simulink model "ball_bouncing"  (R2017b)
settings: Solver=FixedStepAuto  StartTime=0.0  StopTime=10.0  FixedStep=0.001  RelTol=1e-3
values from neighbouring files (symbols this model uses):
  ba = 25    [ball_bouncing_simulation.m]    (also in init_ball_boucing_simulink.m = 1.8)
  d2xa = diff(dxa)    [impact_equations.m]    (also in init_ball_boucing_simulink.m = 0)
  d2xb = diff(dxb)    [impact_equations.m]    (also in init_ball_boucing_simulink.m = 0)
  dxa = diff(xa)    [impact_equations.m]    (also in init_ball_boucing_simulink.m = 0)
  dxb = diff(xb)    [impact_equations.m]    (also in init_ball_boucing_simulink.m = 0)
  g = 9.81    [ball_bouncing_simulation.m]    (also in init_ball_boucing_simulink.m)
  ka = 500    [ball_bouncing_simulation.m]    (also in init_ball_boucing_simulink.m = 25)
  kb = 15000    [ball_bouncing_simulation.m]    (also in init_ball_boucing_simulink.m = 1500)
  ma = 1    [ball_bouncing_simulation.m]    (also in init_ball_boucing_simulink.m = 0.113)
  mb = 0.058    [ball_bouncing_simulation.m]    (also in init_ball_boucing_simulink.m = 0.025)
  r = 0.05    [ball_bouncing_simulation.m]    (also in init_ball_boucing_simulink.m)
  xa = [xa; y(1:idx_end_impact-1,2)]    [ball_bouncing_simulation.m]    (also in init_ball_boucing_simulink.m = 0)
  xb = [xb; y(1:idx_end_impact-1,1)]    [ball_bouncing_simulation.m]    (also in init_ball_boucing_simulink.m = 0.5)
  xv = 0    [ball_bouncing_simulation.m]    (also in init_ball_boucing_simulink.m)
settings Model: Creator=Vincent  LastModifiedBy=Vincent

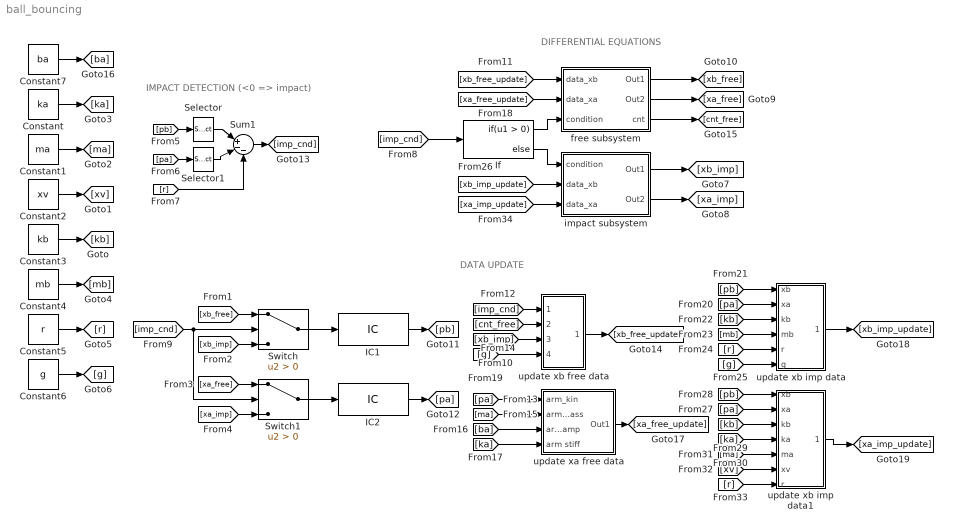
== system ball_bouncing ==
  note: DIFFERENTIAL EQUATIONS
  note: IMPACT DETECTION (<0 => impact)
  note: DATA UPDATE
  Constant : Constant  Value=ka
  Constant1 : Constant  Value=ma
  Constant2 : Constant  Value=xv
  Constant3 : Constant  Value=kb
  Constant4 : Constant  Value=mb
  Constant5 : Constant  Value=r
  Constant6 : Constant  Value=g
  Constant7 : Constant  Value=ba
  IC1 : InitialCondition  Value=[xb;dxb;d2xb]
  IC2 : InitialCondition  Value=[xa;dxa;d2xa]
  If : If
  Selector : Selector  InputPortWidth=3  IndexOptions=Index vector (dialog)  Indices=[1]  OutputSizes=1
  Selector1 : Selector  InputPortWidth=3  IndexOptions=Index vector (dialog)  Indices=[1]  OutputSizes=1
  Sum1 : Sum  Inputs=|+--
  Switch : Switch  Criteria=u2 > Threshold
  Switch1 : Switch  Criteria=u2 > Threshold
  free subsystem : Subsystem
  impact subsystem : Subsystem
  update xa free data : Subsystem
  update xb free data : Subsystem
  update xb imp data : Subsystem
  update xb imp data1 : Subsystem
  wires:
  Constant/1 -> [ka]
  Constant1/1 -> [ma]
  Constant2/1 -> [xv]
  Constant4/1 -> [mb]
  Constant5/1 -> [r]
  Constant6/1 -> [g]
  Constant3/1 -> [kb]
  [imp_cnd] -> If/1
  If/2 -> impact subsystem/1(condition)
  impact subsystem/1(Out1) -> [xb_imp]
  impact subsystem/2(Out2) -> [xa_imp]
  If/1 -> free subsystem/3(condition)
  free subsystem/1(Out1) -> [xb_free]
  free subsystem/2(Out2) -> [xa_free]
  [xb_free] -> Switch/1
  [xb_imp] -> Switch/3
  [xa_free] -> Switch1/1
  [xa_imp] -> Switch1/3
  [pb] -> Selector/1
  Selector/1 -> Sum1/1
  [pa] -> Selector1/1
  Selector1/1 -> Sum1/2
  [r] -> Sum1/3
  Sum1/1 -> [imp_cnd]
  [imp_cnd] -> Switch1/2, Switch/2
  free subsystem/3(cnt) -> [cnt_free]
  [imp_cnd] -> update xb free data/1(In1)
  [cnt_free] -> update xb free data/2(In2)
  [xb_imp] -> update xb free data/3(In3)
  update xb free data/1(Out1) -> [xb_free_update]
  [xb_free_update] -> free subsystem/1(data_xb)
  [pa] -> update xa free data/1(arm_kin)
  [ma] -> update xa free data/2(arm mass)
  [ba] -> update xa free data/3(arm damp)
  [ka] -> update xa free data/4(arm stiff)
  Constant7/1 -> [ba]
  update xa free data/1(Out1) -> [xa_free_update]
  [xa_free_update] -> free subsystem/2(data_xa)
  [g] -> update xb free data/4(In4)
  [pa] -> update xb imp data/2(xa)
  [pb] -> update xb imp data/1(xb)
  [kb] -> update xb imp data/3(kb)
  [mb] -> update xb imp data/4(mb)
  [r] -> update xb imp data/5(r)
  [g] -> update xb imp data/6(g)
  update xb imp data/1(Out1) -> [xb_imp_update]
  [xb_imp_update] -> impact subsystem/2(data_xb)
  update xb imp data1/1(Out1) -> [xa_imp_update]
  [xv] -> update xb imp data1/6(xv)
  [ma] -> update xb imp data1/5(ma)
  [ka] -> update xb imp data1/4(ka)
  [kb] -> update xb imp data1/3(kb)
  [pb] -> update xb imp data1/1(xb)
  [pa] -> update xb imp data1/2(xa)
  [r] -> update xb imp data1/7(r)
  [xa_imp_update] -> impact subsystem/3(data_xa)
  IC2/1 -> [pa]
  Switch/1 -> IC1/1
  IC1/1 -> [pb]
  Switch1/1 -> IC2/1

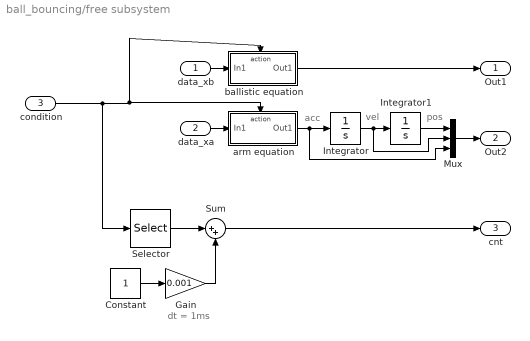
== system ball_bouncing/free subsystem ==
  note: dt = 1ms
  note: acc
  note: pos
  note: vel
  data_xb : Inport
  data_xa : Inport  Port=2
  condition : Inport  Port=3
  Constant : Constant
  Gain : Gain  Gain=0.001
  Integrator : Integrator
  Integrator1 : Integrator
  Mux : Mux  Inputs=3
  Selector : Selector  InputPortWidth=4  IndexOptions=Index vector (dialog)  Indices=[1]  OutputSizes=1
  Sum : Sum  Inputs=|++
  arm equation : Subsystem  TreatAsAtomicUnit=on
  ballistic equation : Subsystem  TreatAsAtomicUnit=on
  Out1 : Outport
  Out2 : Outport  Port=2
  cnt : Outport  Port=3
  wires:
  arm equation/1(Out1) -> Mux/3, Integrator/1
  Integrator/1 -> Mux/2, Integrator1/1
  ballistic equation/1(Out1) -> Out1/1
  condition/1 -> Selector/1, ballistic equation/Action, arm equation/Action
  data_xb/1 -> ballistic equation/1(In1)
  data_xa/1 -> arm equation/1(In1)
  Integrator1/1 -> Mux/1
  Mux/1 -> Out2/1
  Selector/1 -> Sum/1
  Sum/1 -> cnt/1
  Constant/1 -> Gain/1
  Gain/1 -> Sum/2

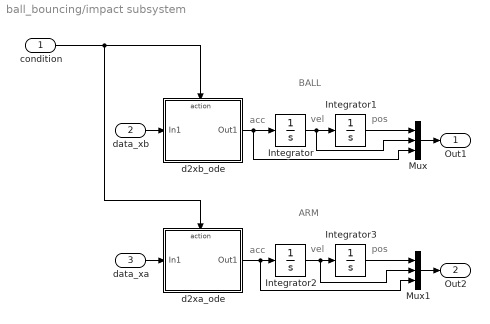
== system ball_bouncing/impact subsystem ==
  note: acc
  note: vel
  note: pos
  note: BALL
  note: acc
  note: vel
  note: pos
  note: ARM
  condition : Inport
  data_xb : Inport  Port=2
  data_xa : Inport  Port=3
  Integrator{,1..3} (4 alike) : Integrator
  Mux : Mux  Inputs=3
  Mux1 : Mux  Inputs=3
  d2xa_ode : Subsystem  TreatAsAtomicUnit=on
  d2xb_ode : Subsystem  TreatAsAtomicUnit=on
  Out1 : Outport
  Out2 : Outport  Port=2
  wires:
  data_xb/1 -> d2xb_ode/1(In1)
  data_xa/1 -> d2xa_ode/1(In1)
  d2xb_ode/1(Out1) -> Mux/3, Integrator/1
  Integrator2/1 -> Mux1/2, Integrator3/1
  d2xa_ode/1(Out1) -> Mux1/3, Integrator2/1
  condition/1 -> d2xb_ode/Action, d2xa_ode/Action
  Integrator/1 -> Mux/2, Integrator1/1
  Mux/1 -> Out1/1
  Integrator1/1 -> Mux/1
  Mux1/1 -> Out2/1
  Integrator3/1 -> Mux1/1

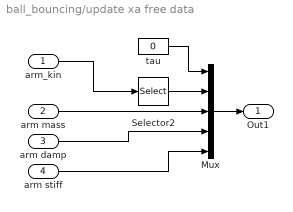
== system ball_bouncing/update xa free data ==
  arm_kin : Inport
  arm mass : Inport  Port=2
  arm damp : Inport  Port=3
  arm stiff : Inport  Port=4
  Mux : Mux  Inputs=5
  Selector2 : Selector  InputPortWidth=3  IndexOptions=Index vector (dialog)  Indices=[1 2]  OutputSizes=1
  tau : Constant  Value=0
  Out1 : Outport
  wires:
  Mux/1 -> Out1/1
  Selector2/1 -> Mux/2
  tau/1 -> Mux/1
  arm_kin/1 -> Selector2/1
  arm mass/1 -> Mux/3
  arm damp/1 -> Mux/4
  arm stiff/1 -> Mux/5

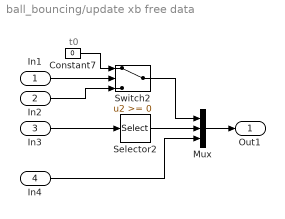
== system ball_bouncing/update xb free data ==
  note: t0
  In1 : Inport
  In2 : Inport  Port=2
  In3 : Inport  Port=3
  In4 : Inport  Port=4
  Constant7 : Constant  Value=0
  Mux : Mux  Inputs=3
  Selector2 : Selector  InputPortWidth=3  IndexOptions=Index vector (dialog)  Indices=[1 2]  OutputSizes=1
  Switch2 : Switch
  Out1 : Outport
  wires:
  In1/1 -> Switch2/2
  Constant7/1 -> Switch2/1
  In3/1 -> Selector2/1
  Mux/1 -> Out1/1
  In2/1 -> Switch2/3
  Selector2/1 -> Mux/2
  In4/1 -> Mux/3
  Switch2/1 -> Mux/1

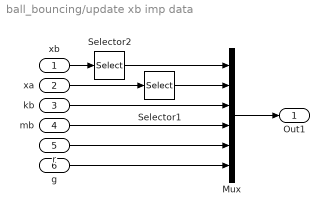
== system ball_bouncing/update xb imp data ==
  xb : Inport
  xa : Inport  Port=2
  kb : Inport  Port=3
  mb : Inport  Port=4
  r : Inport  Port=5
  g : Inport  Port=6
  Mux : Mux  Inputs=6
  Selector1 : Selector  InputPortWidth=3  IndexOptions=Index vector (dialog)  Indices=[1]  OutputSizes=1
  Selector2 : Selector  InputPortWidth=3  IndexOptions=Index vector (dialog)  Indices=[1]  OutputSizes=1
  Out1 : Outport
  wires:
  Mux/1 -> Out1/1
  xb/1 -> Selector2/1
  xa/1 -> Selector1/1
  Selector2/1 -> Mux/1
  Selector1/1 -> Mux/2
  kb/1 -> Mux/3
  mb/1 -> Mux/4
  r/1 -> Mux/5
  g/1 -> Mux/6

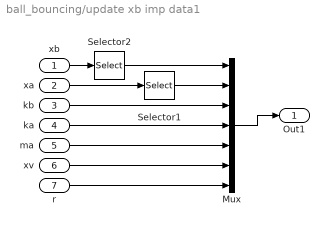
== system ball_bouncing/update xb imp data1 ==
  xb : Inport
  xa : Inport  Port=2
  kb : Inport  Port=3
  ka : Inport  Port=4
  ma : Inport  Port=5
  xv : Inport  Port=6
  r : Inport  Port=7
  Mux : Mux  Inputs=7
  Selector1 : Selector  InputPortWidth=3  IndexOptions=Index vector (dialog)  Indices=[1]  OutputSizes=1
  Selector2 : Selector  InputPortWidth=3  IndexOptions=Index vector (dialog)  Indices=[1]  OutputSizes=1
  Out1 : Outport
  wires:
  xv/1 -> Mux/6
  ma/1 -> Mux/5
  ka/1 -> Mux/4
  kb/1 -> Mux/3
  Selector1/1 -> Mux/2
  Selector2/1 -> Mux/1
  xa/1 -> Selector1/1
  xb/1 -> Selector2/1
  Mux/1 -> Out1/1
  r/1 -> Mux/7

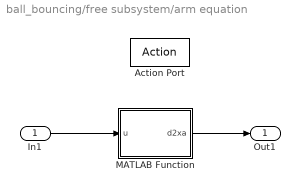
== system ball_bouncing/free subsystem/arm equation ==
  In1 : Inport
  Action Port : ActionPort  ActionType=then
  MATLAB Function : MATLAB Function  TreatAsAtomicUnit=on
  Out1 : Outport
  wires:
  MATLAB Function/1(d2xa) -> Out1/1
  In1/1 -> MATLAB Function/1(u)

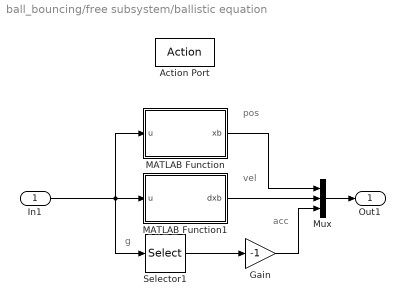
== system ball_bouncing/free subsystem/ballistic equation ==
  note: pos
  note: g
  note: vel
  note: acc
  In1 : Inport
  Action Port : ActionPort  ActionType=then
  Gain : Gain  Gain=-1
  MATLAB Function : MATLAB Function  TreatAsAtomicUnit=on
  MATLAB Function1 : MATLAB Function  TreatAsAtomicUnit=on
  Mux : Mux  Inputs=3
  Selector1 : Selector  InputPortWidth=4  IndexOptions=Index vector (dialog)  Indices=[4]  OutputSizes=1
  Out1 : Outport
  wires:
  In1/1 -> MATLAB Function/1(u), Selector1/1, MATLAB Function1/1(u)
  Selector1/1 -> Gain/1
  MATLAB Function/1(xb) -> Mux/1
  MATLAB Function1/1(dxb) -> Mux/2
  Gain/1 -> Mux/3
  Mux/1 -> Out1/1

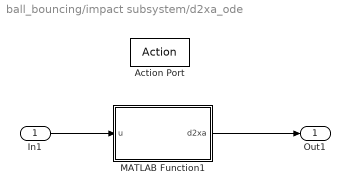
== system ball_bouncing/impact subsystem/d2xa_ode ==
  In1 : Inport
  Action Port : ActionPort  ActionType=else
  MATLAB Function1 : MATLAB Function  TreatAsAtomicUnit=on
  Out1 : Outport
  wires:
  MATLAB Function1/1(d2xa) -> Out1/1
  In1/1 -> MATLAB Function1/1(u)

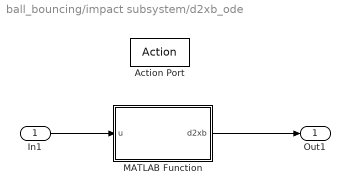
== system ball_bouncing/impact subsystem/d2xb_ode ==
  In1 : Inport
  Action Port : ActionPort  ActionType=else
  MATLAB Function : MATLAB Function  TreatAsAtomicUnit=on
  Out1 : Outport
  wires:
  In1/1 -> MATLAB Function/1(u)
  MATLAB Function/1(d2xb) -> Out1/1

== matlab function ball_bouncing/impact subsystem/d2xa_ode/MATLAB Function1 ==
  data: u input; d2xa output
function d2xa = d2xa_ode(u)

    xb = u(1);
    xa = u(2);
    
    kb = u(3);
    ka = u(4);
    ma = u(5);
    
    xv = u(6);
    r = u(7);

    d2xa = (-ka*(xa - xv) + kb*(xb - xa - r))/ma;

== matlab function ball_bouncing/impact subsystem/d2xb_ode/MATLAB Function ==
  data: u input; d2xb output
function d2xb = d2xb_ode(u)

    xb = u(1);
    xa = u(2);
    
    kb = u(3);
    mb = u(4);
    r = u(5);
    g = u(6);

    d2xb = (-kb*(xb - xa - r) - mb * g)/mb;

== matlab function ball_bouncing/free subsystem/ballistic equation/MATLAB Function ==
  data: u input; xb output
function xb = ballistic_eq(u)

    t = u(1);
    vb0 = u(2);
    h0 = u(3);
    g = u(4);

    xb = -0.5*g*t^2 + vb0*t + h0;

== matlab function ball_bouncing/free subsystem/arm equation/MATLAB Function ==
  data: u input; d2xa output
function d2xa = arm_eq(u)
    
    tau = u(1);
    xa = u(2);
    dxa = u(3);
    ma = u(4);
    ba = u(5);
    ka = u(6);

    d2xa = (tau - ba * dxa - ka * xa)/ma;

== matlab function ball_bouncing/free subsystem/ballistic equation/MATLAB Function1 ==
  data: u input; dxb output
function dxb = ballistic_eq_vel(u)

    t = u(1);
    vb0 = u(2);
    g = u(4);

    dxb = -g*t + vb0;
